simulink model "RealTimeControl"  (R2020b)
settings: Solver=FixedStepDiscrete  StartTime=0.0  StopTime=10.0  FixedStep=0.01  RelTol=1e-3  EnableMultiTasking=on
values from neighbouring files (symbols this model uses):
  Nu = X(5)    [LoadParameters.m]
  Nx = X(1:4)    [LoadParameters.m]
  Ts = 1e-2    (= 0.01)    [LoadParameters.m]
undefined symbols (not defined in the file or in its folder): DiscIntNeverNeededParam, drv, gbox, lqr_integral, lqr_nominal, sens, stvar_est, wheel
libraries: BalRobTbx_baselib x9
settings Model: SILPILModeSetting=veronly  ExtModeTrigDuration=2  Creator=pellizzar1  LastModifiedBy=pellizzar1
settings OptimizationCC: EnhancedBackFolding=on  PassReuseOutputArgsAs=Individual arguments  ZeroExternalMemoryAtStartup=off  ZeroInternalMemoryAtStartup=off  MaxStackSize=64  OptimizeBlockOrder=speed  DifferentSizesBufferReuse=on  OptimizationCustomize=off  EfficientTunableParamExpr=on
settings DebuggingCC: ParameterTunabilityLossMsg=error
settings HardwareCC: ProdBitPerInt=16  ProdBitPerPointer=16  ProdBitPerSizeT=16  ProdBitPerPtrDiffT=16  ProdLargestAtomicFloat=None  ProdWordSize=8  ProdHWDeviceType=Atmel->AVR
settings SFSimCC: MATLABDynamicMemAlloc=off
settings RTWCC: Description=Embedded Coder  SystemTargetFile=ert.tlc  HardwareBoard=Arduino Mega 2560  TemplateMakefile=ert_default_tmf  Toolchain=Arduino AVR  BuildConfiguration=Faster Runs
settings CodeAppCC: ForceParamTrailComments=on  IgnoreCustomStorageClasses=off  OperatorAnnotations=on  SimulinkDataObjDesc=on  SFDataObjDesc=on  InsertBlockDesc=on
settings ERTTargetCC: SupportContinuousTime=on  SupportVariableSizeSignals=on  ExtModeStaticAllocSize=2048

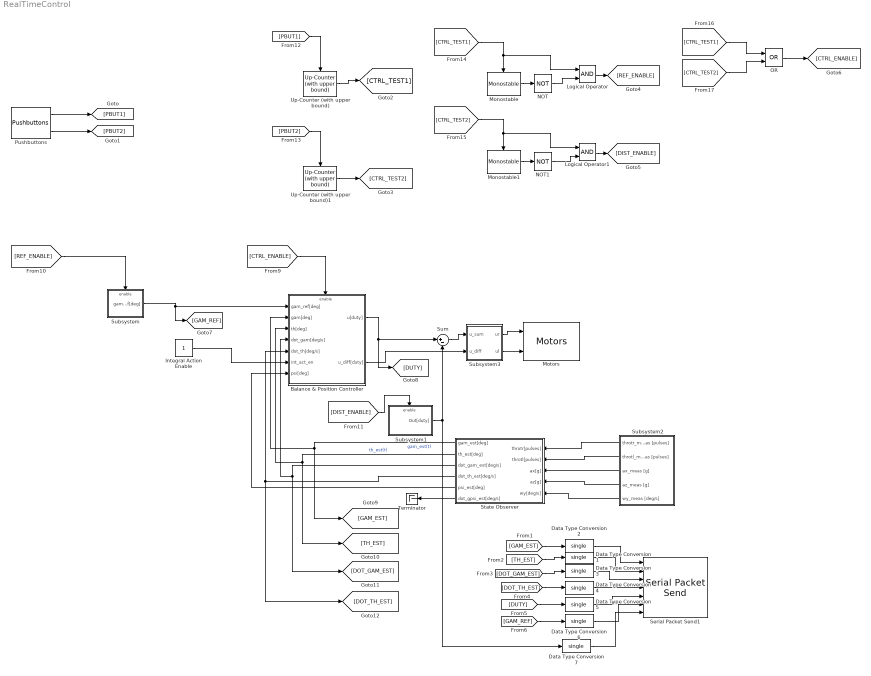
== system RealTimeControl ==
  Balance & Position Controller : Subsystem
  Data Type Conversion{1..7} (7 alike) : DataTypeConversion  OutDataTypeStr=single
  Integral Action Enable : Constant
  Logical Operator : Logic  AllPortsSameDT=off  OutDataTypeStr=boolean
  Logical Operator1 : Logic  AllPortsSameDT=off  OutDataTypeStr=boolean
  Monostable : BalRobTbx_baselib/Utilities/Monostable  Tp=1
      settings: SourceProductName=Balancing Robot Toolbox
  Monostable1 : BalRobTbx_baselib/Utilities/Monostable  Tp=1
      settings: SourceProductName=Balancing Robot Toolbox
  Motors : BalRobTbx_baselib/Outputs/Motors
      settings: SourceProductName=Balancing Robot Toolbox
  NOT : Logic  Operator=NOT  AllPortsSameDT=off  OutDataTypeStr=boolean
  NOT1 : Logic  Operator=NOT  AllPortsSameDT=off  OutDataTypeStr=boolean
  OR : Logic  Operator=OR  AllPortsSameDT=off  OutDataTypeStr=boolean
  Pushbuttons : BalRobTbx_baselib/Inputs/Pushbuttons
      settings: SourceProductName=Balancing Robot Toolbox
  Serial Packet Send1 : BalRobTbx_baselib/Communication/Serial Packet Send  serialLinkOpt=Bluetooth  baudRateOpt=38400  waitHostTxCmd=on  txStartCmd=65  txStopCmd=66  packetSpec={'single','single','single','single','single','single','single'}  cobsEncoded=on  nullTerminated=on  showEnablePort=off
      settings: SourceProductName=Balancing Robot Toolbox
  State Observer : Subsystem
  Subsystem : Subsystem
  Subsystem1 : Subsystem
  Subsystem2 : Subsystem
  Subsystem3 : Subsystem
  Sum : Sum  Inputs=|+-
  Terminator : Terminator
  Up-Counter (with upper bound) : BalRobTbx_baselib/Utilities/Up-Counter (with upper bound)  CMAX=10  C0=0
      settings: SourceProductName=Balancing Robot Toolbox
  Up-Counter (with upper bound)1 : BalRobTbx_baselib/Utilities/Up-Counter (with upper bound)  CMAX=10  C0=0
      settings: SourceProductName=Balancing Robot Toolbox
  wires:
  Pushbuttons/1 -> [PBUT1]
  Pushbuttons/2 -> [PBUT2]
  Integral Action Enable/1 -> Balance & Position Controller/6(int_act_en)
  State Observer/4(dot_th_est[deg/s]) -> [DOT_TH_EST], Balance & Position Controller/5(dot_th[deg/s])
  State Observer/2(th_est[deg]) -> [TH_EST], Balance & Position Controller/3(th[deg])  "th_est(t)"
  State Observer/1(gam_est[deg]) -> [GAM_EST], Balance & Position Controller/2(gam[deg])  "gam_est(t)"
  State Observer/3(dot_gam_est[deg/s]) -> [DOT_GAM_EST], Balance & Position Controller/4(dot_gam[deg/s])
  [CTRL_ENABLE] -> Balance & Position Controller/Enable
  Subsystem/1(gam_ref[deg]) -> [GAM_REF], Balance & Position Controller/1(gam_ref[deg])
  [REF_ENABLE] -> Subsystem/Enable
  Balance & Position Controller/1(u[duty]) -> Sum/1, [DUTY]
  Subsystem1/1(Out[duty]) -> Data Type Conversion7/1, Sum/2
  [DIST_ENABLE] -> Subsystem1/Enable
  Subsystem2/3(ax_meas [g]) -> State Observer/3(ax[g])
  Subsystem2/4(az_meas [g]) -> State Observer/4(az[g])
  Subsystem2/5(wy_meas [deg/s]) -> State Observer/5(wy[deg/s])
  [PBUT1] -> Up-Counter (with upper bound)/Trigger
  Up-Counter (with upper bound)/1 -> [CTRL_TEST1]
  [PBUT2] -> Up-Counter (with upper bound)1/Trigger
  Up-Counter (with upper bound)1/1 -> [CTRL_TEST2]
  [CTRL_TEST1] -> Logical Operator/1, Monostable/Enable
  Monostable/1 -> NOT/1
  NOT/1 -> Logical Operator/2
  Logical Operator/1 -> [REF_ENABLE]
  [CTRL_TEST2] -> Logical Operator1/1, Monostable1/Enable
  Logical Operator1/1 -> [DIST_ENABLE]
  NOT1/1 -> Logical Operator1/2
  Monostable1/1 -> NOT1/1
  [CTRL_TEST1] -> OR/1
  [CTRL_TEST2] -> OR/2
  OR/1 -> [CTRL_ENABLE]
  Data Type Conversion2/1 -> Serial Packet Send1/1
  Data Type Conversion1/1 -> Serial Packet Send1/2
  Data Type Conversion3/1 -> Serial Packet Send1/3
  Data Type Conversion4/1 -> Serial Packet Send1/4
  Data Type Conversion5/1 -> Serial Packet Send1/5
  Data Type Conversion6/1 -> Serial Packet Send1/6
  [GAM_EST] -> Data Type Conversion2/1
  [TH_EST] -> Data Type Conversion1/1
  [DOT_GAM_EST] -> Data Type Conversion3/1
  [DOT_TH_EST] -> Data Type Conversion4/1
  [DUTY] -> Data Type Conversion5/1
  [GAM_REF] -> Data Type Conversion6/1
  Data Type Conversion7/1 -> Serial Packet Send1/7
  Sum/1 -> Subsystem3/1(u_sum)
  Subsystem3/1(ur) -> Motors/1
  Subsystem3/2(ul) -> Motors/2
  State Observer/5(psi_est[deg]) -> Balance & Position Controller/7(psi[deg])
  Subsystem2/2(throtl_meas [pulses]) -> State Observer/2(throtl[pulses])
  Subsystem2/1(throtr_meas [pulses]) -> State Observer/1(throtr[pulses])
  State Observer/6(dot_gpsi_est[deg/s]) -> Terminator/1
  Balance & Position Controller/2(u_diff[duty]) -> Subsystem3/2(u_diff)

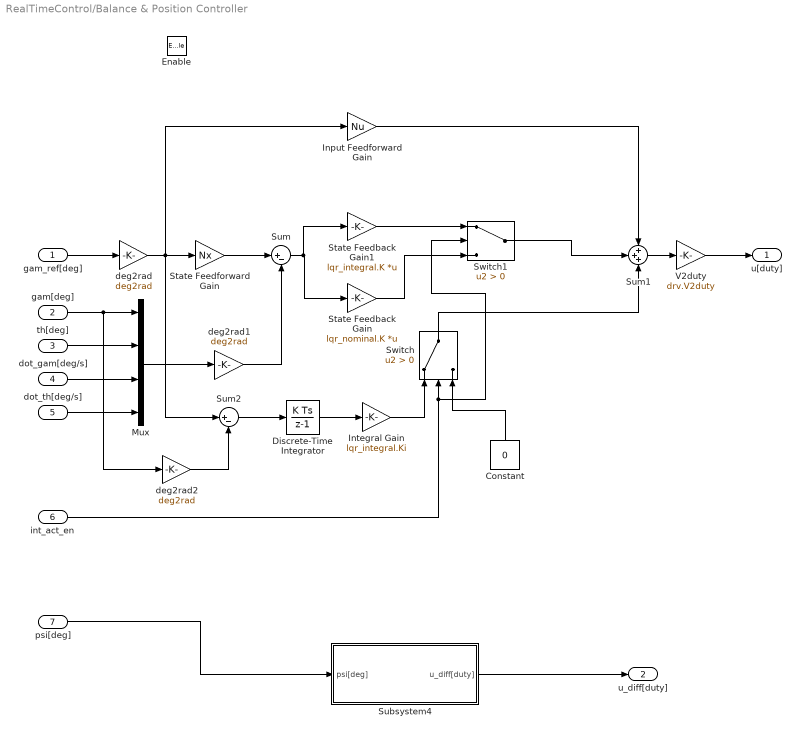
== system RealTimeControl/Balance & Position Controller ==
  gam_ref[deg] : Inport
  gam[deg] : Inport  Port=2
  th[deg] : Inport  Port=3
  dot_gam[deg/s] : Inport  Port=4
  dot_th[deg/s] : Inport  Port=5
  int_act_en : Inport  Port=6
  psi[deg] : Inport  Port=7
  Enable : EnablePort
  Constant : Constant  Value=0
  Discrete-Time Integrator : DiscreteIntegrator  SampleTime=Ts  ICPrevOutput=DiscIntNeverNeededParam  ICPrevScaledInput=DiscIntNeverNeededParam
  Input Feedforward Gain : Gain  Gain=Nu
  Integral Gain : Gain  Gain=lqr_integral.Ki
  Mux : Mux
  State Feedback Gain : Gain  Gain=lqr_nominal.K  Multiplication=Matrix(K*u)
  State Feedback Gain1 : Gain  Gain=lqr_integral.K  Multiplication=Matrix(K*u)
  State Feedforward Gain : Gain  Gain=Nx
  Subsystem4 : Subsystem
  Sum : Sum  Inputs=|+-
  Sum1 : Sum  Inputs=+++
  Sum2 : Sum  Inputs=|+-
  Switch : Switch  Criteria=u2 > Threshold
  Switch1 : Switch  Criteria=u2 > Threshold
  V2duty : Gain  Gain=drv.V2duty
  deg2rad : Gain  Gain=deg2rad
  deg2rad1 : Gain  Gain=deg2rad
  deg2rad2 : Gain  Gain=deg2rad
  u[duty] : Outport  InitialOutput=0
  u_diff[duty] : Outport  Port=2  InitialOutput=0
  wires:
  Mux/1 -> deg2rad1/1
  Sum1/1 -> V2duty/1
  th[deg]/1 -> Mux/2
  deg2rad/1 -> Sum2/1, Input Feedforward Gain/1, State Feedforward Gain/1
  dot_gam[deg/s]/1 -> Mux/3
  Input Feedforward Gain/1 -> Sum1/1
  V2duty/1 -> u[duty]/1
  gam_ref[deg]/1 -> deg2rad/1
  gam[deg]/1 -> deg2rad2/1, Mux/1
  dot_th[deg/s]/1 -> Mux/4
  State Feedforward Gain/1 -> Sum/1
  deg2rad1/1 -> Sum/2
  Sum/1 -> State Feedback Gain1/1, State Feedback Gain/1
  Sum2/1 -> Discrete-Time Integrator/1
  deg2rad2/1 -> Sum2/2
  Discrete-Time Integrator/1 -> Integral Gain/1
  Integral Gain/1 -> Switch/1
  Constant/1 -> Switch/3
  int_act_en/1 -> Switch1/2, Switch/2
  State Feedback Gain/1 -> Switch1/3
  Switch1/1 -> Sum1/2
  State Feedback Gain1/1 -> Switch1/1
  Switch/1 -> Sum1/3
  psi[deg]/1 -> Subsystem4/1(psi[deg])
  Subsystem4/1(u_diff[duty]) -> u_diff[duty]/1

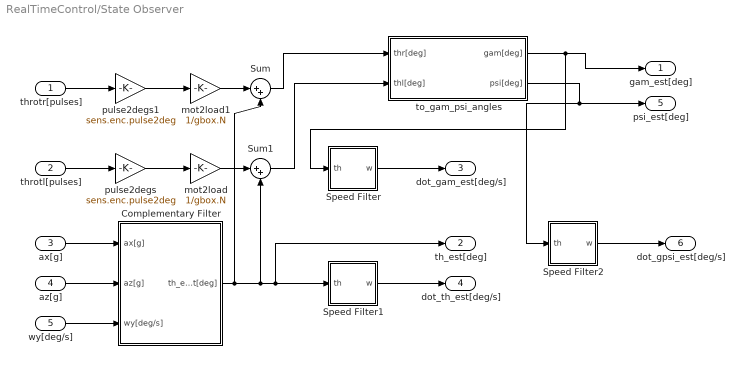
== system RealTimeControl/State Observer ==
  throtr[pulses] : Inport
  throtl[pulses] : Inport  Port=2
  ax[g] : Inport  Port=3
  az[g] : Inport  Port=4
  wy[deg/s] : Inport  Port=5
  Complementary Filter : Subsystem
  Speed Filter : Subsystem
  Speed Filter1 : Subsystem
  Speed Filter2 : Subsystem
  Sum : Sum  Inputs=|++
  Sum1 : Sum  Inputs=|++
  mot2load : Gain  Gain=1/gbox.N
  mot2load1 : Gain  Gain=1/gbox.N
  pulse2degs : Gain  Gain=sens.enc.pulse2deg
  pulse2degs1 : Gain  Gain=sens.enc.pulse2deg
  to_gam_psi_angles : Subsystem
  gam_est[deg] : Outport
  th_est[deg] : Outport  Port=2
  dot_gam_est[deg/s] : Outport  Port=3
  dot_th_est[deg/s] : Outport  Port=4
  psi_est[deg] : Outport  Port=5
  dot_gpsi_est[deg/s] : Outport  Port=6
  wires:
  Complementary Filter/1(th_est[deg]) -> Sum1/2, th_est[deg]/1, Speed Filter1/1(th), Sum/2
  throtl[pulses]/1 -> pulse2degs/1
  ax[g]/1 -> Complementary Filter/1(ax[g])
  az[g]/1 -> Complementary Filter/2(az[g])
  mot2load/1 -> Sum1/1
  wy[deg/s]/1 -> Complementary Filter/3(wy[deg/s])
  Speed Filter/1(w) -> dot_gam_est[deg/s]/1
  Speed Filter1/1(w) -> dot_th_est[deg/s]/1
  pulse2degs/1 -> mot2load/1
  Sum1/1 -> to_gam_psi_angles/2(thl[deg])
  pulse2degs1/1 -> mot2load1/1
  throtr[pulses]/1 -> pulse2degs1/1
  mot2load1/1 -> Sum/1
  Sum/1 -> to_gam_psi_angles/1(thr[deg])
  to_gam_psi_angles/1(gam[deg]) -> Speed Filter/1(th), gam_est[deg]/1
  to_gam_psi_angles/2(psi[deg]) -> psi_est[deg]/1, Speed Filter2/1(th)
  Speed Filter2/1(w) -> dot_gpsi_est[deg/s]/1

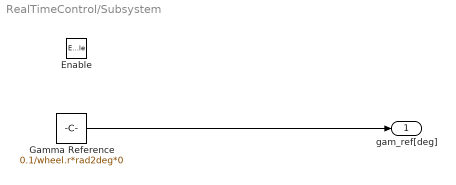
== system RealTimeControl/Subsystem ==
  Enable : EnablePort
  Gamma Reference : Constant  Value=0.1/wheel.r*rad2deg*0
  gam_ref[deg] : Outport
  wires:
  Gamma Reference/1 -> gam_ref[deg]/1

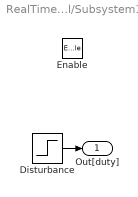
== system RealTimeControl/Subsystem1 ==
  Enable : EnablePort
  Disturbance : Step  Time=10  After=5.0/drv.duty2V  SampleTime=0
  Out[duty] : Outport
  wires:
  Disturbance/1 -> Out[duty]/1

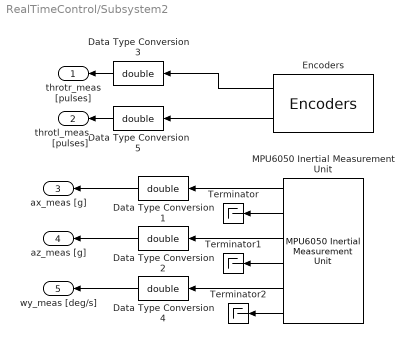
== system RealTimeControl/Subsystem2 ==
  Data Type Conversion{1..5} (5 alike) : DataTypeConversion  OutDataTypeStr=double
  Encoders : BalRobTbx_baselib/Inputs/Encoders
      settings: SourceProductName=Balancing Robot Toolbox
  MPU6050 Inertial Measurement Unit : BalRobTbx_baselib/Inputs/MPU6050 Inertial Measurement Unit
      settings: SourceProductName=Balancing Robot Toolbox
  Terminator : Terminator
  Terminator1 : Terminator
  Terminator2 : Terminator
  throtr_meas [pulses] : Outport
  throtl_meas [pulses] : Outport  Port=2
  ax_meas [g] : Outport  Port=3
  az_meas [g] : Outport  Port=4
  wy_meas [deg/s] : Outport  Port=5
  wires:
  MPU6050 Inertial Measurement Unit/2 -> Terminator/1
  MPU6050 Inertial Measurement Unit/5 -> Data Type Conversion4/1
  Encoders/2 -> Data Type Conversion5/1
  MPU6050 Inertial Measurement Unit/3 -> Data Type Conversion2/1
  MPU6050 Inertial Measurement Unit/4 -> Terminator1/1
  MPU6050 Inertial Measurement Unit/6 -> Terminator2/1
  Encoders/1 -> Data Type Conversion3/1
  MPU6050 Inertial Measurement Unit/1 -> Data Type Conversion1/1
  Data Type Conversion3/1 -> throtr_meas [pulses]/1
  Data Type Conversion4/1 -> wy_meas [deg/s]/1
  Data Type Conversion2/1 -> az_meas [g]/1
  Data Type Conversion1/1 -> ax_meas [g]/1
  Data Type Conversion5/1 -> throtl_meas [pulses]/1

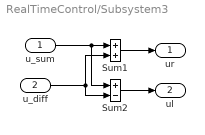
== system RealTimeControl/Subsystem3 ==
  u_sum : Inport
  u_diff : Inport  Port=2
  Sum1 : Sum
  Sum2 : Sum  Inputs=+-
  ur : Outport
  ul : Outport  Port=2
  wires:
  u_sum/1 -> Sum2/1, Sum1/1
  Sum2/1 -> ul/1
  u_diff/1 -> Sum2/2, Sum1/2
  Sum1/1 -> ur/1

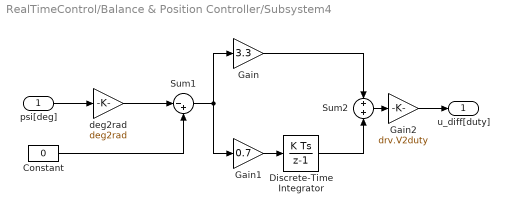
== system RealTimeControl/Balance & Position Controller/Subsystem4 ==
  psi[deg] : Inport
  Constant : Constant  Value=0
  Discrete-Time Integrator : DiscreteIntegrator  SampleTime=Ts  ICPrevOutput=DiscIntNeverNeededParam  ICPrevScaledInput=DiscIntNeverNeededParam
  Gain : Gain  Gain=3.3
  Gain1 : Gain  Gain=0.7
  Gain2 : Gain  Gain=drv.V2duty
  Sum1 : Sum  Inputs=|-+
  Sum2 : Sum  Inputs=+|+
  deg2rad : Gain  Gain=deg2rad
  u_diff[duty] : Outport
  wires:
  Gain2/1 -> u_diff[duty]/1
  Sum1/1 -> Gain1/1, Gain/1
  deg2rad/1 -> Sum1/1
  Gain/1 -> Sum2/1
  psi[deg]/1 -> deg2rad/1
  Sum2/1 -> Gain2/1
  Constant/1 -> Sum1/2
  Discrete-Time Integrator/1 -> Sum2/2
  Gain1/1 -> Discrete-Time Integrator/1

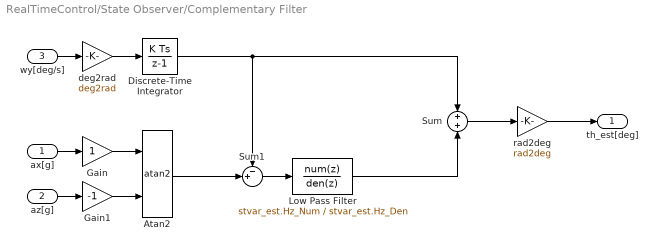
== system RealTimeControl/State Observer/Complementary Filter ==
  ax[g] : Inport
  az[g] : Inport  Port=2
  wy[deg/s] : Inport  Port=3
  Atan2 : Trigonometry  Operator=atan2
  Discrete-Time Integrator : DiscreteIntegrator  SampleTime=Ts  ICPrevOutput=DiscIntNeverNeededParam  ICPrevScaledInput=DiscIntNeverNeededParam
  Gain : Gain
  Gain1 : Gain  Gain=-1
  "Low Pass Filter " : DiscreteTransferFcn  Numerator=stvar_est.Hz_Num  Denominator=stvar_est.Hz_Den
  Sum : Sum  Inputs=+|+
  Sum1 : Sum  Inputs=-+|
  deg2rad : Gain  Gain=deg2rad
  rad2deg : Gain  Gain=rad2deg
  th_est[deg] : Outport
  wires:
  ax[g]/1 -> Gain/1
  deg2rad/1 -> Discrete-Time Integrator/1
  wy[deg/s]/1 -> deg2rad/1
  Atan2/1 -> Sum1/2
  Gain1/1 -> Atan2/2
  Gain/1 -> Atan2/1
  az[g]/1 -> Gain1/1
  rad2deg/1 -> th_est[deg]/1
  Sum/1 -> rad2deg/1
  Discrete-Time Integrator/1 -> Sum1/1, Sum/1
  Sum1/1 -> "Low Pass Filter "/1
  "Low Pass Filter "/1 -> Sum/2

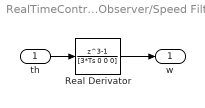
== system RealTimeControl/State Observer/Speed Filter ==
  th : Inport
  Real Derivator : DiscreteTransferFcn  Numerator=[1 0 0 -1]  Denominator=[3*Ts 0 0 0]  SampleTime=Ts
  w : Outport
  wires:
  Real Derivator/1 -> w/1
  th/1 -> Real Derivator/1

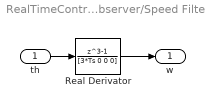
== system RealTimeControl/State Observer/Speed Filter1 ==
  th : Inport
  Real Derivator : DiscreteTransferFcn  Numerator=[1 0 0 -1]  Denominator=[3*Ts 0 0 0]  SampleTime=Ts
  w : Outport
  wires:
  Real Derivator/1 -> w/1
  th/1 -> Real Derivator/1

== system RealTimeControl/State Observer/Speed Filter2 ==
  th : Inport
  Real Derivator : DiscreteTransferFcn  Numerator=[1 0 0 -1]  Denominator=[3*Ts 0 0 0]  SampleTime=Ts
  w : Outport
  wires:
  Real Derivator/1 -> w/1
  th/1 -> Real Derivator/1

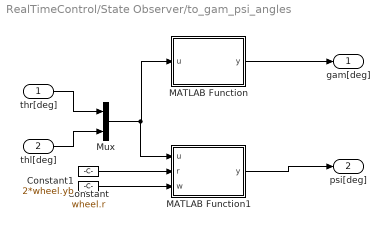
== system RealTimeControl/State Observer/to_gam_psi_angles ==
  thr[deg] : Inport
  thl[deg] : Inport  Port=2
  Constant : Constant  Value=wheel.r
  Constant1 : Constant  Value=2*wheel.yb
  MATLAB Function : MATLAB Function  TreatAsAtomicUnit=on
  MATLAB Function1 : MATLAB Function  TreatAsAtomicUnit=on
  Mux : Mux  Inputs=2
  gam[deg] : Outport
  psi[deg] : Outport  Port=2
  wires:
  thl[deg]/1 -> Mux/2
  Constant1/1 -> MATLAB Function1/3(w)
  thr[deg]/1 -> Mux/1
  MATLAB Function1/1(y) -> psi[deg]/1
  Constant/1 -> MATLAB Function1/2(r)
  Mux/1 -> MATLAB Function1/1(u), MATLAB Function/1(u)
  MATLAB Function/1(y) -> gam[deg]/1

== matlab function RealTimeControl/State Observer/to_gam_psi_angles/MATLAB Function ==
  data: u input; y output
function y = fcn(u)

y = (u(1)+u(2))/2;

== matlab function RealTimeControl/State Observer/to_gam_psi_angles/MATLAB Function1 ==
  data: u input; y output; r input; w input
function y = fcn(u, r, w)

y = r/w*(u(1)-u(2));
